simulink model "UPS_3level_Ttype_Inverter_simplified_ctrl"  (R2012b)
settings: Solver=ode4  StartTime=0.0  StopTime=Tfinal  FixedStep=Ts  MaxStep=1e-5  RelTol=1e-3
values from neighbouring files (symbols this model uses):
  Ts = 1/(1*1e6)    (= 1e-06)    [Run.m]
  Vd = 720    [Run.m]
  VSI = rmfield(VSI, {'IF1', 'IF2', 'FLUXlin1', 'FLUXlin2',      'FLUXnonlin1', 'FLUXnonlin2', 'Lfnonlin'})    [Run.m]
undefined symbols (not defined in the file or in its folder): ADC, CTRL, DiscIntNeverNeededParam, PR, S, UPS
libraries: powerlib x113, simulink_extras x11, powerlib_extras x11, simulink x3
(part 2 of 3)

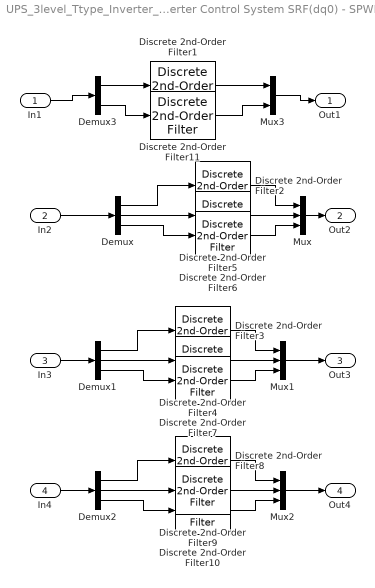
== system UPS_3level_Ttype_Inverter_simplified_ctrl/Output Inverter Control System SRF(dq0) - SPWM /input filter1 ==
  In1 : Inport
  In2 : Inport  Port=2
  In3 : Inport  Port=3
  In4 : Inport  Port=4
  Demux : Demux  Outputs=3
  Demux1 : Demux  Outputs=3
  Demux2 : Demux  Outputs=3
  Demux3 : Demux  Outputs=2
  Discrete 2nd-Order Filter1 : powerlib_extras/Discrete  Control Blocks/Discrete  2nd-Order Filter  FilterType=Lowpass  Fo=25000  Zeta=0.89  Ts=Ts  Initialize=off  Vac_Init=[0.8 -25 60]  Vdc_Init=-0.4  PlotResponse=off  param1=[1 500 1]
  Discrete 2nd-Order Filter{2..10} (9 alike) : powerlib_extras/Discrete  Control Blocks/Discrete  2nd-Order Filter  FilterType=Lowpass  Fo=25e3  Zeta=0.89  Ts=Ts  Initialize=off  Vac_Init=[0.8 -25 60]  Vdc_Init=-0.4  PlotResponse=off  param1=[1 500 1]
  Discrete 2nd-Order Filter11 : powerlib_extras/Discrete  Control Blocks/Discrete  2nd-Order Filter  FilterType=Lowpass  Fo=25000  Zeta=0.89  Ts=Ts  Initialize=off  Vac_Init=[0.8 -25 60]  Vdc_Init=-0.4  PlotResponse=off  param1=[1 500 1]
  Mux : Mux  Inputs=3
  Mux1 : Mux  Inputs=3
  Mux2 : Mux  Inputs=3
  Mux3 : Mux  Inputs=2
  Out1 : Outport
  Out2 : Outport  Port=2
  Out3 : Outport  Port=3
  Out4 : Outport  Port=4
  wires:
  Demux/3 -> Discrete 2nd-Order Filter6/1
  In2/1 -> Demux/1
  Mux/1 -> Out2/1
  Demux/1 -> Discrete 2nd-Order Filter2/1
  Demux/2 -> Discrete 2nd-Order Filter5/1
  Discrete 2nd-Order Filter5/1 -> Mux/2
  Discrete 2nd-Order Filter6/1 -> Mux/3
  Discrete 2nd-Order Filter2/1 -> Mux/1
  Demux1/3 -> Discrete 2nd-Order Filter7/1
  Demux1/1 -> Discrete 2nd-Order Filter3/1
  Demux1/2 -> Discrete 2nd-Order Filter4/1
  Discrete 2nd-Order Filter4/1 -> Mux1/2
  Discrete 2nd-Order Filter7/1 -> Mux1/3
  Discrete 2nd-Order Filter3/1 -> Mux1/1
  Demux2/3 -> Discrete 2nd-Order Filter10/1
  Demux2/1 -> Discrete 2nd-Order Filter8/1
  Demux2/2 -> Discrete 2nd-Order Filter9/1
  Discrete 2nd-Order Filter9/1 -> Mux2/2
  Discrete 2nd-Order Filter10/1 -> Mux2/3
  Discrete 2nd-Order Filter8/1 -> Mux2/1
  Mux2/1 -> Out4/1
  Mux1/1 -> Out3/1
  In3/1 -> Demux1/1
  In4/1 -> Demux2/1
  Demux3/2 -> Discrete 2nd-Order Filter11/1
  Demux3/1 -> Discrete 2nd-Order Filter1/1
  Discrete 2nd-Order Filter1/1 -> Mux3/1
  Discrete 2nd-Order Filter11/1 -> Mux3/2
  Mux3/1 -> Out1/1
  In1/1 -> Demux3/1

== system UPS_3level_Ttype_Inverter_simplified_ctrl/Output filter (Cf2, Lf2)/2phasM1 ==
  Constant2 : Constant  Value=UPS.Lfnonlin
  Data Type Conversion2 : DataTypeConversion  OutDataTypeStr=boolean  SaturateOnIntegerOverflow=on  RndMeth=Zero
  Discrete-Time Integrator : DiscreteIntegrator  gainval=1  SampleTime=Ts  ICPrevOutput=DiscIntNeverNeededParam  ICPrevScaledInput=DiscIntNeverNeededParam
  Lookup Table : Lookup  InputValues=VSI.FLUXnonlin  Table=VSI.IF
  Lookup Table1 : Lookup  InputValues=VSI.FLUXlin  Table=VSI.IF
  Switch2 : Switch  Threshold=1
  if : powerlib/Electrical Sources/Controlled Current Source  Initialize=on  Source_Type=AC  Amplitude=0  Phase=0  Frequency=0  Measurements=None
  vf : powerlib/Measurements/Voltage Measurement  PhasorSimulation=off  OutputType=Complex  PSBequivalent=0
  x : PMIOPort  Port=1  Side=Left
  y : PMIOPort  Port=2  Side=Right
  wires:
  vf/1 -> Discrete-Time Integrator/1
  Discrete-Time Integrator/1 -> Lookup Table/1, Lookup Table1/1
  Data Type Conversion2/1 -> Switch2/2
  Constant2/1 -> Data Type Conversion2/1
  Lookup Table1/1 -> Switch2/3
  Lookup Table/1 -> Switch2/1
  Switch2/1 -> if/1
  connections:
  if/RConn1 -- y/RConn1 -- vf/LConn2
  x/RConn1 -- vf/LConn1 -- if/LConn1

== system UPS_3level_Ttype_Inverter_simplified_ctrl/Output filter (Cf2, Lf2)/2phasM2 ==
  Constant2 : Constant  Value=UPS.Lfnonlin
  Data Type Conversion2 : DataTypeConversion  OutDataTypeStr=boolean  SaturateOnIntegerOverflow=on  RndMeth=Zero
  Discrete-Time Integrator : DiscreteIntegrator  gainval=1  SampleTime=Ts  ICPrevOutput=DiscIntNeverNeededParam  ICPrevScaledInput=DiscIntNeverNeededParam
  Lookup Table : Lookup  InputValues=VSI.FLUXnonlin  Table=VSI.IF
  Lookup Table1 : Lookup  InputValues=VSI.FLUXlin  Table=VSI.IF
  Switch2 : Switch  Threshold=1
  if : powerlib/Electrical Sources/Controlled Current Source  Initialize=on  Source_Type=AC  Amplitude=0  Phase=0  Frequency=0  Measurements=None
  vf : powerlib/Measurements/Voltage Measurement  PhasorSimulation=off  OutputType=Complex  PSBequivalent=0
  x : PMIOPort  Port=1  Side=Left
  y : PMIOPort  Port=2  Side=Right
  wires:
  vf/1 -> Discrete-Time Integrator/1
  Discrete-Time Integrator/1 -> Lookup Table/1, Lookup Table1/1
  Data Type Conversion2/1 -> Switch2/2
  Constant2/1 -> Data Type Conversion2/1
  Lookup Table1/1 -> Switch2/3
  Lookup Table/1 -> Switch2/1
  Switch2/1 -> if/1
  connections:
  if/RConn1 -- y/RConn1 -- vf/LConn2
  x/RConn1 -- vf/LConn1 -- if/LConn1

== system UPS_3level_Ttype_Inverter_simplified_ctrl/Output filter (Cf2, Lf2)/2phasM8 ==
  Constant2 : Constant  Value=UPS.Lfnonlin
  Data Type Conversion2 : DataTypeConversion  OutDataTypeStr=boolean  SaturateOnIntegerOverflow=on  RndMeth=Zero
  Discrete-Time Integrator : DiscreteIntegrator  gainval=1  SampleTime=Ts  ICPrevOutput=DiscIntNeverNeededParam  ICPrevScaledInput=DiscIntNeverNeededParam
  Lookup Table : Lookup  InputValues=VSI.FLUXnonlin  Table=VSI.IF
  Lookup Table1 : Lookup  InputValues=VSI.FLUXlin  Table=VSI.IF
  Switch2 : Switch  Threshold=1
  if : powerlib/Electrical Sources/Controlled Current Source  Initialize=on  Source_Type=AC  Amplitude=0  Phase=0  Frequency=0  Measurements=None
  vf : powerlib/Measurements/Voltage Measurement  PhasorSimulation=off  OutputType=Complex  PSBequivalent=0
  x : PMIOPort  Port=1  Side=Left
  y : PMIOPort  Port=2  Side=Right
  wires:
  vf/1 -> Discrete-Time Integrator/1
  Discrete-Time Integrator/1 -> Lookup Table/1, Lookup Table1/1
  Data Type Conversion2/1 -> Switch2/2
  Constant2/1 -> Data Type Conversion2/1
  Lookup Table1/1 -> Switch2/3
  Lookup Table/1 -> Switch2/1
  Switch2/1 -> if/1
  connections:
  if/RConn1 -- y/RConn1 -- vf/LConn2
  x/RConn1 -- vf/LConn1 -- if/LConn1

== system UPS_3level_Ttype_Inverter_simplified_ctrl/Output Inverter Control System SRF(dq0) - SPWM /3p PLL/va, vb ==
  Vm* [pu] : Inport
  "wrt* [deg] " : Inport  Port=2
  va* = Vm*cos(wrt)* : Subsystem
  vb* = Vm*sin(wrt)* : Subsystem
  cos(wrt)* : Outport
  sin(wrt)* : Outport  Port=2
  wires:
  Vm* [pu]/1 -> va* = Vm*cos(wrt)*/1(Vm [pu]), vb* = Vm*sin(wrt)*/1(Vm [pu])
  va* = Vm*cos(wrt)*/1(va) -> cos(wrt)*/1
  vb* = Vm*sin(wrt)*/1(vb) -> sin(wrt)*/1
  "wrt* [deg] "/1 -> vb* = Vm*sin(wrt)*/2(wrt [deg]), va* = Vm*cos(wrt)*/2(wrt [deg])

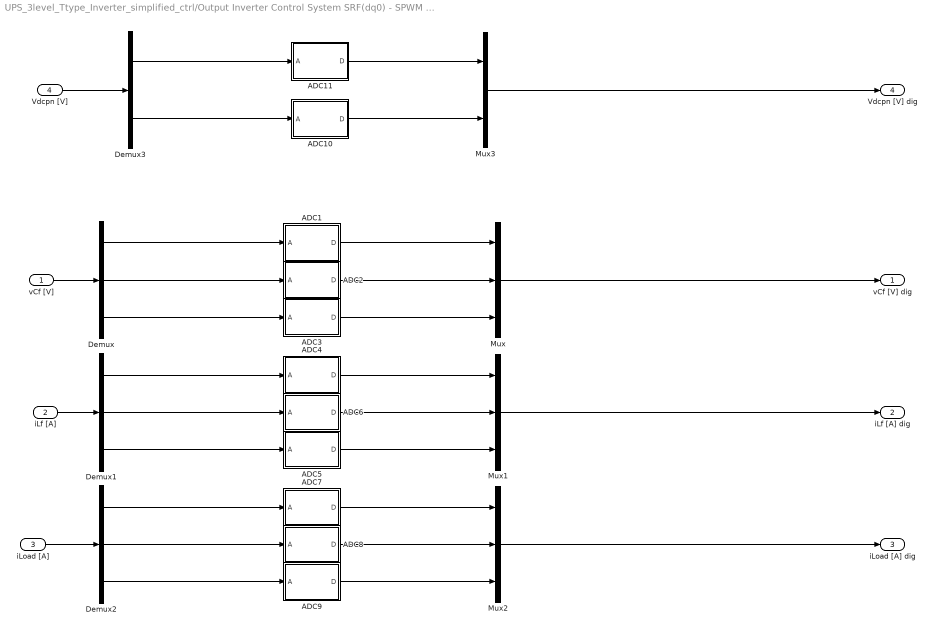
== system UPS_3level_Ttype_Inverter_simplified_ctrl/Output Inverter Control System SRF(dq0) - SPWM /SPWM (Treg)2/ ADC System (Tinp//2) ==
  vCf [V] : Inport
  iLf [A] : Inport  Port=2
  iLoad [A] : Inport  Port=3
  Vdcpn [V] : Inport  Port=4
  ADC1 : Subsystem
  ADC10 : Subsystem
  ADC11 : Subsystem
  ADC2 : Subsystem
  ADC3 : Subsystem
  ADC4 : Subsystem
  ADC5 : Subsystem
  ADC6 : Subsystem
  ADC7 : Subsystem
  ADC8 : Subsystem
  ADC9 : Subsystem
  Demux : Demux  Outputs=3
  Demux1 : Demux  Outputs=3
  Demux2 : Demux  Outputs=3
  Demux3 : Demux  Outputs=2
  Mux : Mux  Inputs=3
  Mux1 : Mux  Inputs=3
  Mux2 : Mux  Inputs=3
  Mux3 : Mux  Inputs=2
  vCf [V] dig : Outport
  iLf [A] dig : Outport  Port=2
  iLoad [A] dig : Outport  Port=3
  Vdcpn [V] dig : Outport  Port=4
  wires:
  Demux/1 -> ADC1/1(A)
  Demux/2 -> ADC2/1(A)
  Demux/3 -> ADC3/1(A)
  ADC1/1(D) -> Mux/1
  ADC2/1(D) -> Mux/2
  ADC3/1(D) -> Mux/3
  Demux1/1 -> ADC4/1(A)
  Demux1/2 -> ADC6/1(A)
  Demux1/3 -> ADC5/1(A)
  ADC4/1(D) -> Mux1/1
  ADC6/1(D) -> Mux1/2
  ADC5/1(D) -> Mux1/3
  Demux2/1 -> ADC7/1(A)
  Demux2/2 -> ADC8/1(A)
  Demux2/3 -> ADC9/1(A)
  ADC7/1(D) -> Mux2/1
  ADC8/1(D) -> Mux2/2
  ADC9/1(D) -> Mux2/3
  vCf [V]/1 -> Demux/1
  iLf [A]/1 -> Demux1/1
  iLoad [A]/1 -> Demux2/1
  Mux/1 -> vCf [V] dig/1
  Mux1/1 -> iLf [A] dig/1
  Mux2/1 -> iLoad [A] dig/1
  Mux3/1 -> Vdcpn [V] dig/1
  ADC10/1(D) -> Mux3/2
  Demux3/2 -> ADC10/1(A)
  Demux3/1 -> ADC11/1(A)
  ADC11/1(D) -> Mux3/1
  Vdcpn [V]/1 -> Demux3/1

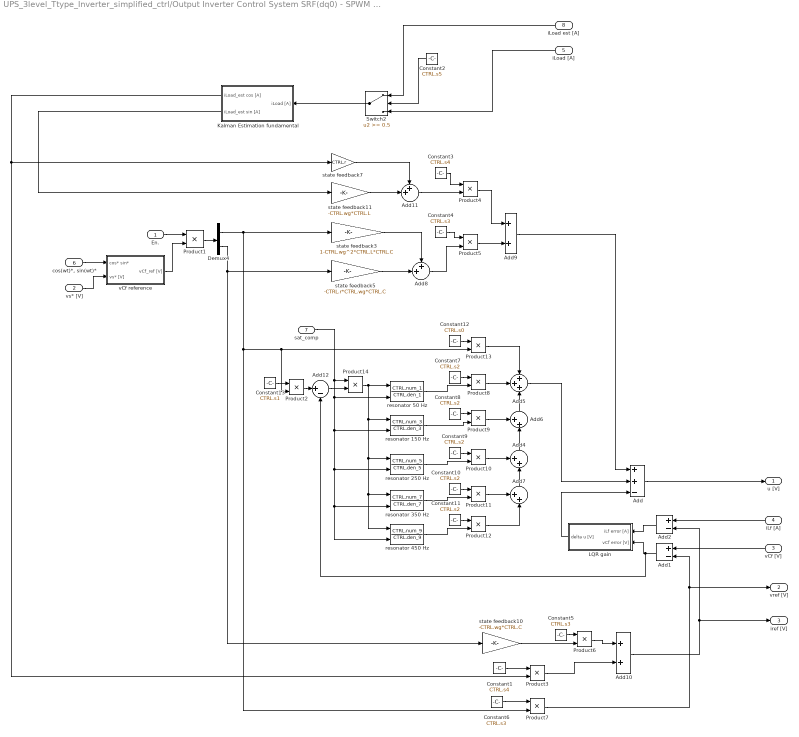
== system UPS_3level_Ttype_Inverter_simplified_ctrl/Output Inverter Control System SRF(dq0) - SPWM /SPWM (Treg)2/controller ph a1 ==
  En. : Inport
  vs* [V] : Inport  Port=2
  vCf [V] : Inport  Port=3
  iLf [A] : Inport  Port=4
  iLoad [A] : Inport  Port=5
  "cos(wt)*, sin(wt)*" : Inport  Port=6
  sat_comp : Inport  Port=7
  iLoad est [A] : Inport  Port=8
  Add : Sum  Inputs=++-
  Add1 : Sum  Inputs=+-
  Add10 : Sum
  Add{4,6..8,11} (5 alike) : Sum  Inputs=++|
  Add12 : Sum  Inputs=|+-
  Add2 : Sum  Inputs=+-
  Add5 : Sum  Inputs=+++
  Add9 : Sum
  Constant1 : Constant  Value=CTRL.s4
  Constant{7..11} (5 alike) : Constant  Value=CTRL.s2
  Constant12 : Constant  Value=CTRL.s0
  Constant13 : Constant  Value=CTRL.s1
  Constant2 : Constant  Value=CTRL.s5
  Constant3 : Constant  Value=CTRL.s4
  Constant4 : Constant  Value=CTRL.s3
  Constant5 : Constant  Value=CTRL.s3
  Constant6 : Constant  Value=CTRL.s3
  Demux4 : Demux  Outputs=2
  Kalman Estimation fundamental : Subsystem
  LQR gain : Subsystem
  Product{1..14} (14 alike) : Product  RndMeth=Zero
  Switch2 : Switch  Threshold=0.5
  resonator 150 Hz : DiscreteTransferFcn  Numerator=CTRL.num_3  Denominator=CTRL.den_3  ExternalReset=Falling
      settings: InputPortMap=u0,r7
  resonator 250 Hz : DiscreteTransferFcn  Numerator=CTRL.num_5  Denominator=CTRL.den_5  ExternalReset=Falling
      settings: InputPortMap=u0,r7
  resonator 350 Hz : DiscreteTransferFcn  Numerator=CTRL.num_7  Denominator=CTRL.den_7  ExternalReset=Falling
      settings: InputPortMap=u0,r7
  resonator 450 Hz : DiscreteTransferFcn  Numerator=CTRL.num_9  Denominator=CTRL.den_9  ExternalReset=Falling
      settings: InputPortMap=u0,r7
  resonator 50 Hz : DiscreteTransferFcn  Numerator=CTRL.num_1  Denominator=CTRL.den_1  ExternalReset=Falling
      settings: InputPortMap=u0,r7
  state feedback10 : Gain  Gain=-CTRL.wg*CTRL.C
  state feedback11 : Gain  Gain=-CTRL.wg*CTRL.L
  state feedback3 : Gain  Gain=1-CTRL.wg^2*CTRL.L*CTRL.C
  state feedback5 : Gain  Gain=-CTRL.r*CTRL.wg*CTRL.C
  state feedback7 : Gain  Gain=CTRL.r
  vCf reference : Subsystem
  u [V] : Outport
  vref [V] : Outport  Port=2
  iref [V] : Outport  Port=3
  wires:
  vs* [V]/1 -> vCf reference/2(vs* [V])
  "cos(wt)*, sin(wt)*"/1 -> vCf reference/1(cos* sin*)
  En./1 -> Product1/1
  vCf reference/1(vCf_ref [V]) -> Product1/2
  Add2/1 -> LQR gain/1(iLf error [A])
  LQR gain/1(delta u [V]) -> Add/3
  Product1/1 -> Demux4/1
  iLf [A]/1 -> Add2/1
  Add/1 -> u [V]/1
  vCf [V]/1 -> Add1/1
  Add10/1 -> iref [V]/1, Add2/2
  state feedback10/1 -> Product6/2
  Kalman Estimation fundamental/1(iLoad_est cos [A]) -> Product3/2, state feedback7/1
  Demux4/2 -> state feedback5/1, state feedback10/1
  Demux4/1 -> state feedback3/1, Product2/2, Product13/2, Product7/2
  Kalman Estimation fundamental/2(iLoad_est sin [A]) -> state feedback11/1
  Add9/1 -> Add/1
  Add11/1 -> Product4/2
  state feedback7/1 -> Add11/1
  state feedback5/1 -> Add8/2
  state feedback11/1 -> Add11/2
  state feedback3/1 -> Add8/1
  Add8/1 -> Product5/2
  Add5/1 -> Add/2
  Add7/1 -> Add4/2
  Add4/1 -> Add6/2
  Add6/1 -> Add5/3
  Product14/1 -> resonator 450 Hz/1, resonator 350 Hz/1, resonator 250 Hz/1, resonator 150 Hz/1, resonator 50 Hz/1
  Add1/1 -> Add12/2, LQR gain/2(vCf error [V])
  Constant2/1 -> Switch2/2
  Switch2/1 -> Kalman Estimation fundamental/1(iLoad [A])
  iLoad est [A]/1 -> Switch2/1
  iLoad [A]/1 -> Switch2/3
  Constant1/1 -> Product3/1
  Product3/1 -> Add10/2
  Constant3/1 -> Product4/1
  Product4/1 -> Add9/1
  Constant4/1 -> Product5/1
  Product5/1 -> Add9/2
  Constant5/1 -> Product6/1
  Product6/1 -> Add10/1
  Constant6/1 -> Product7/1
  Product7/1 -> Add1/2, vref [V]/1
  Constant7/1 -> Product8/1
  Constant8/1 -> Product9/1
  Constant9/1 -> Product10/1
  Constant10/1 -> Product11/1
  Constant11/1 -> Product12/1
  Product8/1 -> Add5/2
  Product9/1 -> Add6/1
  Product10/1 -> Add4/1
  Product11/1 -> Add7/1
  Product12/1 -> Add7/2
  resonator 450 Hz/1 -> Product12/2
  resonator 50 Hz/1 -> Product8/2
  resonator 150 Hz/1 -> Product9/2
  resonator 250 Hz/1 -> Product10/2
  resonator 350 Hz/1 -> Product11/2
  Constant12/1 -> Product13/1
  Product13/1 -> Add5/1
  Constant13/1 -> Product2/1
  Product2/1 -> Add12/1
  Add12/1 -> Product14/2
  sat_comp/1 -> Product14/1, resonator 450 Hz/2, resonator 350 Hz/2, resonator 250 Hz/2, resonator 150 Hz/2, resonator 50 Hz/2

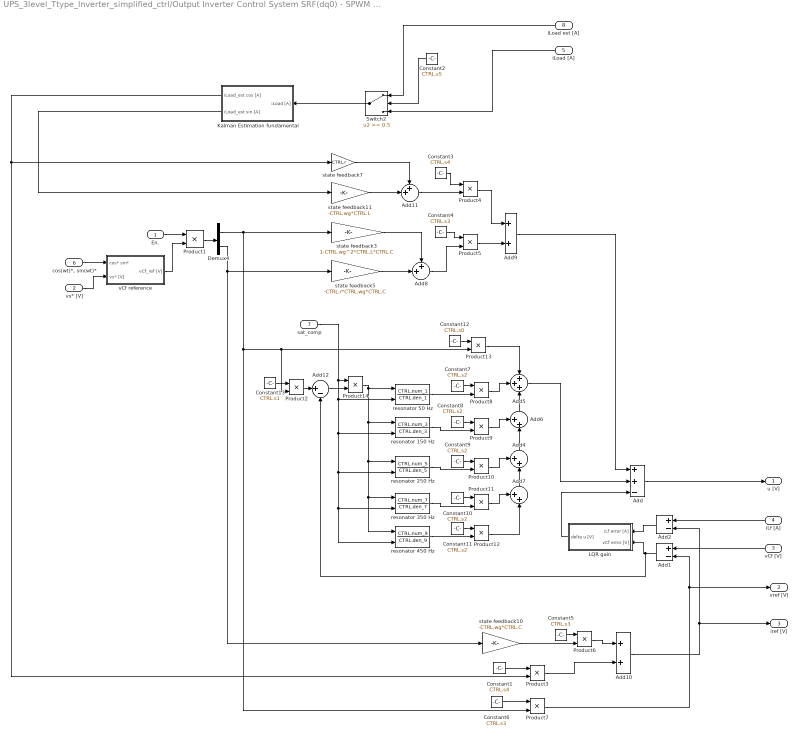
== system UPS_3level_Ttype_Inverter_simplified_ctrl/Output Inverter Control System SRF(dq0) - SPWM /SPWM (Treg)2/controller ph a2 ==
  En. : Inport
  vs* [V] : Inport  Port=2
  vCf [V] : Inport  Port=3
  iLf [A] : Inport  Port=4
  iLoad [A] : Inport  Port=5
  "cos(wt)*, sin(wt)*" : Inport  Port=6
  sat_comp : Inport  Port=7
  iLoad est [A] : Inport  Port=8
  Add : Sum  Inputs=++-
  Add1 : Sum  Inputs=+-
  Add10 : Sum
  Add{4,6..8,11} (5 alike) : Sum  Inputs=++|
  Add12 : Sum  Inputs=|+-
  Add2 : Sum  Inputs=+-
  Add5 : Sum  Inputs=+++
  Add9 : Sum
  Constant1 : Constant  Value=CTRL.s4
  Constant{7..11} (5 alike) : Constant  Value=CTRL.s2
  Constant12 : Constant  Value=CTRL.s0
  Constant13 : Constant  Value=CTRL.s1
  Constant2 : Constant  Value=CTRL.s5
  Constant3 : Constant  Value=CTRL.s4
  Constant4 : Constant  Value=CTRL.s3
  Constant5 : Constant  Value=CTRL.s3
  Constant6 : Constant  Value=CTRL.s3
  Demux4 : Demux  Outputs=2
  Kalman Estimation fundamental : Subsystem
  LQR gain : Subsystem
  Product{1..14} (14 alike) : Product  RndMeth=Zero
  Switch2 : Switch  Threshold=0.5
  resonator 150 Hz : DiscreteTransferFcn  Numerator=CTRL.num_3  Denominator=CTRL.den_3  ExternalReset=Falling
      settings: InputPortMap=u0,r7
  resonator 250 Hz : DiscreteTransferFcn  Numerator=CTRL.num_5  Denominator=CTRL.den_5  ExternalReset=Falling
      settings: InputPortMap=u0,r7
  resonator 350 Hz : DiscreteTransferFcn  Numerator=CTRL.num_7  Denominator=CTRL.den_7  ExternalReset=Falling
      settings: InputPortMap=u0,r7
  resonator 450 Hz : DiscreteTransferFcn  Numerator=CTRL.num_9  Denominator=CTRL.den_9  ExternalReset=Falling
      settings: InputPortMap=u0,r7
  resonator 50 Hz : DiscreteTransferFcn  Numerator=CTRL.num_1  Denominator=CTRL.den_1  ExternalReset=Falling
      settings: InputPortMap=u0,r7
  state feedback10 : Gain  Gain=-CTRL.wg*CTRL.C
  state feedback11 : Gain  Gain=-CTRL.wg*CTRL.L
  state feedback3 : Gain  Gain=1-CTRL.wg^2*CTRL.L*CTRL.C
  state feedback5 : Gain  Gain=-CTRL.r*CTRL.wg*CTRL.C
  state feedback7 : Gain  Gain=CTRL.r
  vCf reference : Subsystem
  u [V] : Outport
  vref [V] : Outport  Port=2
  iref [V] : Outport  Port=3
  wires:
  Add12/1 -> Product14/2
  sat_comp/1 -> resonator 450 Hz/2, resonator 350 Hz/2, resonator 250 Hz/2, resonator 150 Hz/2, resonator 50 Hz/2, Product14/1
  Product2/1 -> Add12/1
  Constant13/1 -> Product2/1
  Product13/1 -> Add5/1
  Constant12/1 -> Product13/1
  resonator 350 Hz/1 -> Product11/2
  resonator 250 Hz/1 -> Product10/2
  resonator 150 Hz/1 -> Product9/2
  resonator 50 Hz/1 -> Product8/2
  resonator 450 Hz/1 -> Product12/2
  Product12/1 -> Add7/2
  Product11/1 -> Add7/1
  Product10/1 -> Add4/1
  Product9/1 -> Add6/1
  Product8/1 -> Add5/2
  Constant11/1 -> Product12/1
  Constant10/1 -> Product11/1
  Constant9/1 -> Product10/1
  Constant8/1 -> Product9/1
  Constant7/1 -> Product8/1
  Product7/1 -> vref [V]/1, Add1/2
  Constant6/1 -> Product7/1
  Product6/1 -> Add10/1
  Constant5/1 -> Product6/1
  Product5/1 -> Add9/2
  Constant4/1 -> Product5/1
  Product4/1 -> Add9/1
  Constant3/1 -> Product4/1
  Product3/1 -> Add10/2
  Constant1/1 -> Product3/1
  iLoad [A]/1 -> Switch2/3
  iLoad est [A]/1 -> Switch2/1
  Switch2/1 -> Kalman Estimation fundamental/1(iLoad [A])
  Constant2/1 -> Switch2/2
  Add1/1 -> LQR gain/2(vCf error [V]), Add12/2
  Product14/1 -> resonator 50 Hz/1, resonator 150 Hz/1, resonator 250 Hz/1, resonator 350 Hz/1, resonator 450 Hz/1
  Add6/1 -> Add5/3
  Add4/1 -> Add6/2
  Add7/1 -> Add4/2
  Add5/1 -> Add/2
  Add8/1 -> Product5/2
  state feedback3/1 -> Add8/1
  state feedback11/1 -> Add11/2
  state feedback5/1 -> Add8/2
  state feedback7/1 -> Add11/1
  Add11/1 -> Product4/2
  Add9/1 -> Add/1
  Kalman Estimation fundamental/2(iLoad_est sin [A]) -> state feedback11/1
  Demux4/1 -> Product7/2, Product13/2, Product2/2, state feedback3/1
  Demux4/2 -> state feedback10/1, state feedback5/1
  Kalman Estimation fundamental/1(iLoad_est cos [A]) -> state feedback7/1, Product3/2
  state feedback10/1 -> Product6/2
  Add10/1 -> iref [V]/1, Add2/2
  vCf [V]/1 -> Add1/1
  Add/1 -> u [V]/1
  iLf [A]/1 -> Add2/1
  Product1/1 -> Demux4/1
  LQR gain/1(delta u [V]) -> Add/3
  Add2/1 -> LQR gain/1(iLf error [A])
  vCf reference/1(vCf_ref [V]) -> Product1/2
  En./1 -> Product1/1
  "cos(wt)*, sin(wt)*"/1 -> vCf reference/1(cos* sin*)
  vs* [V]/1 -> vCf reference/2(vs* [V])

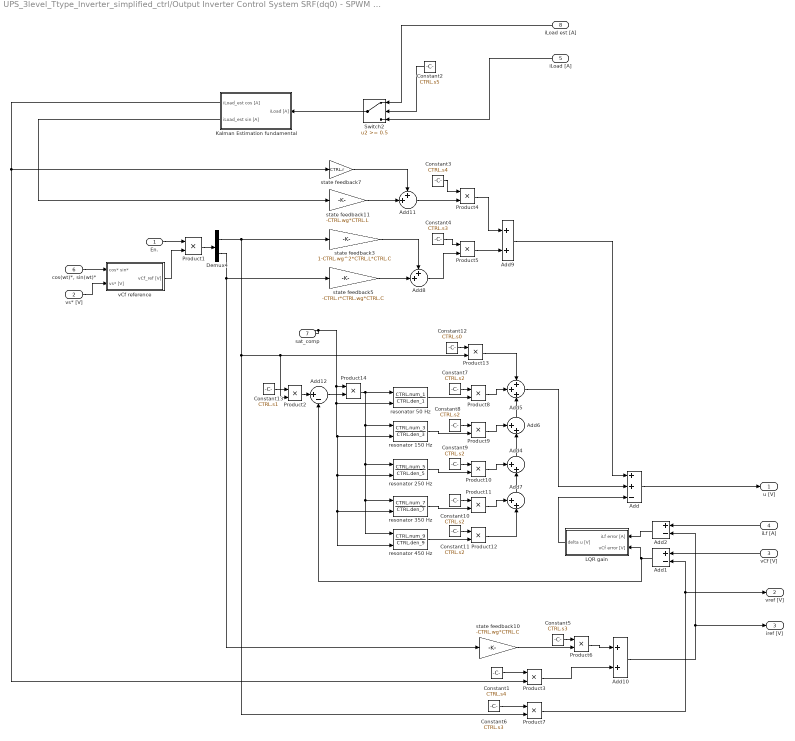
== system UPS_3level_Ttype_Inverter_simplified_ctrl/Output Inverter Control System SRF(dq0) - SPWM /SPWM (Treg)2/controller ph a3 ==
  En. : Inport
  vs* [V] : Inport  Port=2
  vCf [V] : Inport  Port=3
  iLf [A] : Inport  Port=4
  iLoad [A] : Inport  Port=5
  "cos(wt)*, sin(wt)*" : Inport  Port=6
  sat_comp : Inport  Port=7
  iLoad est [A] : Inport  Port=8
  Add : Sum  Inputs=++-
  Add1 : Sum  Inputs=+-
  Add10 : Sum
  Add{4,6..8,11} (5 alike) : Sum  Inputs=++|
  Add12 : Sum  Inputs=|+-
  Add2 : Sum  Inputs=+-
  Add5 : Sum  Inputs=+++
  Add9 : Sum
  Constant1 : Constant  Value=CTRL.s4
  Constant{7..11} (5 alike) : Constant  Value=CTRL.s2
  Constant12 : Constant  Value=CTRL.s0
  Constant13 : Constant  Value=CTRL.s1
  Constant2 : Constant  Value=CTRL.s5
  Constant3 : Constant  Value=CTRL.s4
  Constant4 : Constant  Value=CTRL.s3
  Constant5 : Constant  Value=CTRL.s3
  Constant6 : Constant  Value=CTRL.s3
  Demux4 : Demux  Outputs=2
  Kalman Estimation fundamental : Subsystem
  LQR gain : Subsystem
  Product{1..14} (14 alike) : Product  RndMeth=Zero
  Switch2 : Switch  Threshold=0.5
  resonator 150 Hz : DiscreteTransferFcn  Numerator=CTRL.num_3  Denominator=CTRL.den_3  ExternalReset=Falling
      settings: InputPortMap=u0,r7
  resonator 250 Hz : DiscreteTransferFcn  Numerator=CTRL.num_5  Denominator=CTRL.den_5  ExternalReset=Falling
      settings: InputPortMap=u0,r7
  resonator 350 Hz : DiscreteTransferFcn  Numerator=CTRL.num_7  Denominator=CTRL.den_7  ExternalReset=Falling
      settings: InputPortMap=u0,r7
  resonator 450 Hz : DiscreteTransferFcn  Numerator=CTRL.num_9  Denominator=CTRL.den_9  ExternalReset=Falling
      settings: InputPortMap=u0,r7
  resonator 50 Hz : DiscreteTransferFcn  Numerator=CTRL.num_1  Denominator=CTRL.den_1  ExternalReset=Falling
      settings: InputPortMap=u0,r7
  state feedback10 : Gain  Gain=-CTRL.wg*CTRL.C
  state feedback11 : Gain  Gain=-CTRL.wg*CTRL.L
  state feedback3 : Gain  Gain=1-CTRL.wg^2*CTRL.L*CTRL.C
  state feedback5 : Gain  Gain=-CTRL.r*CTRL.wg*CTRL.C
  state feedback7 : Gain  Gain=CTRL.r
  vCf reference : Subsystem
  u [V] : Outport
  vref [V] : Outport  Port=2
  iref [V] : Outport  Port=3
  wires:
  vs* [V]/1 -> vCf reference/2(vs* [V])
  "cos(wt)*, sin(wt)*"/1 -> vCf reference/1(cos* sin*)
  En./1 -> Product1/1
  vCf reference/1(vCf_ref [V]) -> Product1/2
  Add2/1 -> LQR gain/1(iLf error [A])
  LQR gain/1(delta u [V]) -> Add/3
  Product1/1 -> Demux4/1
  iLf [A]/1 -> Add2/1
  Add/1 -> u [V]/1
  vCf [V]/1 -> Add1/1
  Add10/1 -> iref [V]/1, Add2/2
  state feedback10/1 -> Product6/2
  Kalman Estimation fundamental/1(iLoad_est cos [A]) -> Product3/2, state feedback7/1
  Demux4/2 -> state feedback5/1, state feedback10/1
  Demux4/1 -> state feedback3/1, Product2/2, Product13/2, Product7/2
  Kalman Estimation fundamental/2(iLoad_est sin [A]) -> state feedback11/1
  Add9/1 -> Add/1
  Add11/1 -> Product4/2
  state feedback7/1 -> Add11/1
  state feedback5/1 -> Add8/2
  state feedback11/1 -> Add11/2
  state feedback3/1 -> Add8/1
  Add8/1 -> Product5/2
  Add5/1 -> Add/2
  Add7/1 -> Add4/2
  Add4/1 -> Add6/2
  Add6/1 -> Add5/3
  Product14/1 -> resonator 450 Hz/1, resonator 350 Hz/1, resonator 250 Hz/1, resonator 150 Hz/1, resonator 50 Hz/1
  Add1/1 -> Add12/2, LQR gain/2(vCf error [V])
  Constant2/1 -> Switch2/2
  Switch2/1 -> Kalman Estimation fundamental/1(iLoad [A])
  iLoad est [A]/1 -> Switch2/1
  iLoad [A]/1 -> Switch2/3
  Constant1/1 -> Product3/1
  Product3/1 -> Add10/2
  Constant3/1 -> Product4/1
  Product4/1 -> Add9/1
  Constant4/1 -> Product5/1
  Product5/1 -> Add9/2
  Constant5/1 -> Product6/1
  Product6/1 -> Add10/1
  Constant6/1 -> Product7/1
  Product7/1 -> Add1/2, vref [V]/1
  Constant7/1 -> Product8/1
  Constant8/1 -> Product9/1
  Constant9/1 -> Product10/1
  Constant10/1 -> Product11/1
  Constant11/1 -> Product12/1
  Product8/1 -> Add5/2
  Product9/1 -> Add6/1
  Product10/1 -> Add4/1
  Product11/1 -> Add7/1
  Product12/1 -> Add7/2
  resonator 450 Hz/1 -> Product12/2
  resonator 50 Hz/1 -> Product8/2
  resonator 150 Hz/1 -> Product9/2
  resonator 250 Hz/1 -> Product10/2
  resonator 350 Hz/1 -> Product11/2
  Constant12/1 -> Product13/1
  Product13/1 -> Add5/1
  Constant13/1 -> Product2/1
  Product2/1 -> Add12/1
  sat_comp/1 -> resonator 450 Hz/2, resonator 350 Hz/2, resonator 250 Hz/2, resonator 150 Hz/2, resonator 50 Hz/2, Product14/1
  Add12/1 -> Product14/2

== system UPS_3level_Ttype_Inverter_simplified_ctrl/Output Inverter Control System SRF(dq0) - SPWM /SPWM (Treg)2/iLoad estimator ==
  iLf [A] : Inport
  vCf [V] : Inport  Port=2
  Add : Sum  Inputs=+-
  Add1 : Sum  Inputs=+-
  Discrete Transfer Fcn7 : DiscreteTransferFcn  Numerator=CTRL.num_lp  Denominator=CTRL.den_lp
  Gain1 : Gain  Gain=VSI.Cf/VSI.Treg
  Unit Delay : UnitDelay  SampleTime=-1
  iLoad_est [A] : Outport
  wires:
  Discrete Transfer Fcn7/1 -> iLoad_est [A]/1
  iLf [A]/1 -> Add/1
  Add1/1 -> Gain1/1
  Unit Delay/1 -> Add1/2
  vCf [V]/1 -> Add1/1, Unit Delay/1
  Gain1/1 -> Add/2
  Add/1 -> Discrete Transfer Fcn7/1

== system UPS_3level_Ttype_Inverter_simplified_ctrl/Output Inverter Control System SRF(dq0) - SPWM /SPWM (Treg)2/iLoad estimator1 ==
  iLf [A] : Inport
  vCf [V] : Inport  Port=2
  Add : Sum  Inputs=+-
  Add1 : Sum  Inputs=+-
  Discrete Transfer Fcn7 : DiscreteTransferFcn  Numerator=CTRL.num_lp  Denominator=CTRL.den_lp
  Gain1 : Gain  Gain=VSI.Cf/VSI.Treg
  Unit Delay : UnitDelay  SampleTime=-1
  iLoad_est [A] : Outport
  wires:
  Add/1 -> Discrete Transfer Fcn7/1
  Gain1/1 -> Add/2
  vCf [V]/1 -> Unit Delay/1, Add1/1
  Unit Delay/1 -> Add1/2
  Add1/1 -> Gain1/1
  iLf [A]/1 -> Add/1
  Discrete Transfer Fcn7/1 -> iLoad_est [A]/1

== system UPS_3level_Ttype_Inverter_simplified_ctrl/Output Inverter Control System SRF(dq0) - SPWM /SPWM (Treg)2/iLoad estimator2 ==
  iLf [A] : Inport
  vCf [V] : Inport  Port=2
  Add : Sum  Inputs=+-
  Add1 : Sum  Inputs=+-
  Discrete Transfer Fcn7 : DiscreteTransferFcn  Numerator=CTRL.num_lp  Denominator=CTRL.den_lp
  Gain1 : Gain  Gain=VSI.Cf/VSI.Treg
  Unit Delay : UnitDelay  SampleTime=-1
  iLoad_est [A] : Outport
  wires:
  Discrete Transfer Fcn7/1 -> iLoad_est [A]/1
  iLf [A]/1 -> Add/1
  Add1/1 -> Gain1/1
  Unit Delay/1 -> Add1/2
  vCf [V]/1 -> Add1/1, Unit Delay/1
  Gain1/1 -> Add/2
  Add/1 -> Discrete Transfer Fcn7/1

== system UPS_3level_Ttype_Inverter_simplified_ctrl/Output Inverter Control System SRF(dq0) - SPWM /SPWM (Treg)2/phase a signals ==
  vCf [V] : Inport
  iLf [A] : Inport  Port=2
  iLoad [A] : Inport  Port=3
  cos sin : Inport  Port=4
  Demux : Demux  Outputs=3
  Demux1 : Demux  Outputs=3
  Demux2 : Demux  Outputs=3
  Terminator{1..6} (6 alike) : Terminator
  vCf ph a  [V] : Outport
  iLf ph a [A] : Outport  Port=2
  iLoad pha [A] : Outport  Port=3
  "cos, sin" : Outport  Port=4
  wires:
  Demux1/3 -> Terminator4/1
  Demux/3 -> Terminator2/1
  Demux1/2 -> Terminator3/1
  Demux/2 -> Terminator1/1
  vCf [V]/1 -> Demux/1
  iLf [A]/1 -> Demux1/1
  Demux/1 -> vCf ph a  [V]/1
  Demux1/1 -> iLf ph a [A]/1
  Demux2/3 -> Terminator6/1
  Demux2/2 -> Terminator5/1
  iLoad [A]/1 -> Demux2/1
  Demux2/1 -> iLoad pha [A]/1
  cos sin/1 -> "cos, sin"/1

== system UPS_3level_Ttype_Inverter_simplified_ctrl/Output Inverter Control System SRF(dq0) - SPWM /SPWM (Treg)2/phase b signals ==
  vCf [V] : Inport
  iLf [A] : Inport  Port=2
  iLoad [A] : Inport  Port=3
  cos sin : Inport  Port=4
  Add : Sum
  Add1 : Sum
  Demux : Demux  Outputs=3
  Demux1 : Demux  Outputs=3
  Demux2 : Demux  Outputs=3
  Demux3 : Demux  Outputs=2
  Gain1 : Gain  Gain=cos(2*pi/3)
  Gain2 : Gain  Gain=sin(2*pi/3)
  Gain3 : Gain  Gain=cos(2*pi/3)
  Gain4 : Gain  Gain=-sin(2*pi/3)
  Mux2 : Mux  Inputs=2
  Terminator{1..6} (6 alike) : Terminator
  vCf ph b  [V] : Outport
  iLf ph b [A] : Outport  Port=2
  iLoad ph b [A] : Outport  Port=3
  cos sin rot -120 deg : Outport  Port=4
  wires:
  Demux1/2 -> iLf ph b [A]/1
  Demux/2 -> vCf ph b  [V]/1
  iLf [A]/1 -> Demux1/1
  vCf [V]/1 -> Demux/1
  Demux/1 -> Terminator1/1
  Demux1/1 -> Terminator3/1
  Demux/3 -> Terminator2/1
  Demux1/3 -> Terminator4/1
  Demux2/3 -> Terminator6/1
  Demux2/1 -> Terminator5/1
  cos sin/1 -> Demux3/1
  Demux3/1 -> Gain1/1, Gain4/1
  Demux3/2 -> Gain2/1, Gain3/1
  Gain1/1 -> Add/1
  Gain2/1 -> Add/2
  Add/1 -> Mux2/1
  Mux2/1 -> cos sin rot -120 deg/1
  Add1/1 -> Mux2/2
  Gain4/1 -> Add1/1
  Gain3/1 -> Add1/2
  iLoad [A]/1 -> Demux2/1
  Demux2/2 -> iLoad ph b [A]/1

== system UPS_3level_Ttype_Inverter_simplified_ctrl/Output Inverter Control System SRF(dq0) - SPWM /SPWM (Treg)2/phase c signals ==
  vCf [V] : Inport
  iLf [A] : Inport  Port=2
  iLoad [A] : Inport  Port=3
  cos sin : Inport  Port=4
  Add : Sum
  Add1 : Sum
  Demux : Demux  Outputs=3
  Demux1 : Demux  Outputs=3
  Demux2 : Demux  Outputs=3
  Demux3 : Demux  Outputs=2
  Gain1 : Gain  Gain=cos(2*pi/3)
  Gain2 : Gain  Gain=-sin(2*pi/3)
  Gain3 : Gain  Gain=cos(2*pi/3)
  Gain4 : Gain  Gain=sin(2*pi/3)
  Mux2 : Mux  Inputs=2
  Terminator{1..6} (6 alike) : Terminator
  vCf ph c  [V] : Outport
  iLf ph c [A] : Outport  Port=2
  iLoad ph c [A] : Outport  Port=3
  cos sin rot +120 deg : Outport  Port=4
  wires:
  Demux1/2 -> Terminator4/1
  Demux/2 -> Terminator2/1
  Demux1/1 -> Terminator3/1
  Demux/1 -> Terminator1/1
  vCf [V]/1 -> Demux/1
  iLf [A]/1 -> Demux1/1
  Demux/3 -> vCf ph c  [V]/1
  Demux1/3 -> iLf ph c [A]/1
  Demux2/1 -> Terminator6/1
  Demux2/2 -> Terminator5/1
  Gain3/1 -> Add1/2
  Gain4/1 -> Add1/1
  Add1/1 -> Mux2/2
  Mux2/1 -> cos sin rot +120 deg/1
  Add/1 -> Mux2/1
  Gain2/1 -> Add/2
  Gain1/1 -> Add/1
  Demux3/2 -> Gain3/1, Gain2/1
  Demux3/1 -> Gain4/1, Gain1/1
  cos sin/1 -> Demux3/1
  iLoad [A]/1 -> Demux2/1
  Demux2/3 -> iLoad ph c [A]/1

== system UPS_3level_Ttype_Inverter_simplified_ctrl/Output Inverter Control System SRF(dq0) - SPWM /SPWM (Treg)2/va, vb1 ==
  u [pu] : Inport
  Add : Sum  Inputs=+-
  Constant : Constant  Value=-1
  Constant1 : Constant
  Constant2 : Constant
  Data Type Conversion : DataTypeConversion  OutDataTypeStr=double
  Logical Operator : Logic  Operator=OR  AllPortsSameDT=off  OutDataTypeStr=boolean
  Relational Operator1 : RelationalOperator  Operator=<  OutDataTypeStr=boolean
  Relational Operator2 : RelationalOperator  Operator=>  OutDataTypeStr=boolean
  sat_comp : Outport
  wires:
  u [pu]/1 -> Relational Operator2/1, Relational Operator1/1
  Constant1/1 -> Relational Operator2/2
  Constant/1 -> Relational Operator1/2
  Relational Operator2/1 -> Logical Operator/1
  Relational Operator1/1 -> Logical Operator/2
  Logical Operator/1 -> Data Type Conversion/1
  Data Type Conversion/1 -> Add/2
  Add/1 -> sat_comp/1
  Constant2/1 -> Add/1

== system UPS_3level_Ttype_Inverter_simplified_ctrl/Output Inverter Control System SRF(dq0) - SPWM /SPWM (Treg)2/va, vb2 ==
  u [pu] : Inport
  Add : Sum  Inputs=+-
  Constant : Constant  Value=-1
  Constant1 : Constant
  Constant2 : Constant
  Data Type Conversion : DataTypeConversion  OutDataTypeStr=double
  Logical Operator : Logic  Operator=OR  AllPortsSameDT=off  OutDataTypeStr=boolean
  Relational Operator1 : RelationalOperator  Operator=<  OutDataTypeStr=boolean
  Relational Operator2 : RelationalOperator  Operator=>  OutDataTypeStr=boolean
  sat_comp : Outport
  wires:
  Constant2/1 -> Add/1
  Add/1 -> sat_comp/1
  Data Type Conversion/1 -> Add/2
  Logical Operator/1 -> Data Type Conversion/1
  Relational Operator1/1 -> Logical Operator/2
  Relational Operator2/1 -> Logical Operator/1
  Constant/1 -> Relational Operator1/2
  Constant1/1 -> Relational Operator2/2
  u [pu]/1 -> Relational Operator1/1, Relational Operator2/1

== system UPS_3level_Ttype_Inverter_simplified_ctrl/Output Inverter Control System SRF(dq0) - SPWM /SPWM (Treg)2/va, vb3 ==
  u [pu] : Inport
  Add : Sum  Inputs=+-
  Constant : Constant  Value=-1
  Constant1 : Constant
  Constant2 : Constant
  Data Type Conversion : DataTypeConversion  OutDataTypeStr=double
  Logical Operator : Logic  Operator=OR  AllPortsSameDT=off  OutDataTypeStr=boolean
  Relational Operator1 : RelationalOperator  Operator=<  OutDataTypeStr=boolean
  Relational Operator2 : RelationalOperator  Operator=>  OutDataTypeStr=boolean
  sat_comp : Outport
  wires:
  u [pu]/1 -> Relational Operator2/1, Relational Operator1/1
  Constant1/1 -> Relational Operator2/2
  Constant/1 -> Relational Operator1/2
  Relational Operator2/1 -> Logical Operator/1
  Relational Operator1/1 -> Logical Operator/2
  Logical Operator/1 -> Data Type Conversion/1
  Data Type Conversion/1 -> Add/2
  Add/1 -> sat_comp/1
  Constant2/1 -> Add/1

== system UPS_3level_Ttype_Inverter_simplified_ctrl/Output Inverter Control System SRF(dq0) - SPWM /SPWM (Treg)2/va, vb4 ==
  u [V] : Inport
  Vdcpn [V] : Inport  Port=2
  Demux : Demux  Outputs=2
  Divide1 : Product  Inputs=*/
  Gain : Gain  Gain=0.5
  Sum : Sum  Inputs=|++
  u [pu] : Outport
  wires:
  u [V]/1 -> Divide1/1
  Divide1/1 -> u [pu]/1
  Vdcpn [V]/1 -> Demux/1
  Demux/1 -> Sum/1
  Demux/2 -> Sum/2
  Sum/1 -> Gain/1
  Gain/1 -> Divide1/2

== system UPS_3level_Ttype_Inverter_simplified_ctrl/Output Inverter Control System SRF(dq0) - SPWM /SPWM (Treg)2/va, vb5 ==
  u [V] : Inport
  Vdcpn [V] : Inport  Port=2
  Demux : Demux  Outputs=2
  Divide1 : Product  Inputs=*/
  Gain : Gain  Gain=0.5
  Sum : Sum  Inputs=|++
  u [pu] : Outport
  wires:
  u [V]/1 -> Divide1/1
  Divide1/1 -> u [pu]/1
  Vdcpn [V]/1 -> Demux/1
  Demux/1 -> Sum/1
  Demux/2 -> Sum/2
  Sum/1 -> Gain/1
  Gain/1 -> Divide1/2

== system UPS_3level_Ttype_Inverter_simplified_ctrl/Output Inverter Control System SRF(dq0) - SPWM /SPWM (Treg)2/va, vb6 ==
  u [V] : Inport
  Vdcpn [V] : Inport  Port=2
  Demux : Demux  Outputs=2
  Divide1 : Product  Inputs=*/
  Gain : Gain  Gain=0.5
  Sum : Sum  Inputs=|++
  u [pu] : Outport
  wires:
  u [V]/1 -> Divide1/1
  Divide1/1 -> u [pu]/1
  Vdcpn [V]/1 -> Demux/1
  Demux/1 -> Sum/1
  Demux/2 -> Sum/2
  Sum/1 -> Gain/1
  Gain/1 -> Divide1/2

== system UPS_3level_Ttype_Inverter_simplified_ctrl/Output Inverter Control System SRF(dq0) - SPWM /3p PLL/va, vb/va* = Vm*cos(wrt)* ==
  Vm [pu] : Inport
  wrt [deg] : Inport  Port=2
  Fcn1 : Fcn  Expr=(cos(u(1)))
  Product : Product  SaturateOnIntegerOverflow=on  InputSameDT=on  OutDataTypeStr=Inherit: Same as first input
  d2r : Gain  Gain=pi/180  SaturateOnIntegerOverflow=on  OutDataTypeStr=Inherit: Same as input  ParamDataTypeStr=Inherit: Same as input
  va : Outport
  wires:
  d2r/1 -> Fcn1/1
  Fcn1/1 -> Product/1
  Vm [pu]/1 -> Product/2
  Product/1 -> va/1
  wrt [deg]/1 -> d2r/1

== system UPS_3level_Ttype_Inverter_simplified_ctrl/Output Inverter Control System SRF(dq0) - SPWM /3p PLL/va, vb/vb* = Vm*sin(wrt)* ==
  Vm [pu] : Inport
  wrt [deg] : Inport  Port=2
  Fcn1 : Fcn  Expr=(sin(u(1)))
  Product : Product  SaturateOnIntegerOverflow=on  InputSameDT=on  OutDataTypeStr=Inherit: Same as first input
  d2r : Gain  Gain=pi/180  SaturateOnIntegerOverflow=on  OutDataTypeStr=Inherit: Same as input  ParamDataTypeStr=Inherit: Same as input
  vb : Outport
  wires:
  d2r/1 -> Fcn1/1
  Fcn1/1 -> Product/1
  Vm [pu]/1 -> Product/2
  Product/1 -> vb/1
  wrt [deg]/1 -> d2r/1

== system UPS_3level_Ttype_Inverter_simplified_ctrl/Output Inverter Control System SRF(dq0) - SPWM /SPWM (Treg)2/ ADC System (Tinp//2)/ADC1 ==
  A : Inport
  Add1 : Sum  Inputs=+-
  Add2 : Sum
  Add3 : Sum
  Add7 : Sum
  Constant1 : Constant  Value=ADC.Voffset
  Constant2 : Constant  Value=(2^ADC.N)/2
  Data Type Conversion1 : DataTypeConversion  OutDataTypeStr=int16  SaturateOnIntegerOverflow=on  RndMeth=Zero
  Data Type Conversion2 : DataTypeConversion  OutDataTypeStr=double  SaturateOnIntegerOverflow=on  RndMeth=Zero
  Gain : Gain  Gain=ADC.k1vABC
  Gain1 : Gain  Gain=ADC.k2vABC
  Gain2 : Gain  Gain=ADC.Nonlin*((ADC.Vmax - ADC.Vmin)/2^ADC.N)
  Gain3 : Gain  Gain=ADC.Nnoise*((ADC.Vmax - ADC.Vmin)/2^ADC.N)
  Idealized ADC quantizer : simulink_extras/Additional Discrete/Idealized ADC quantizer  NumberOfConverterBits=ADC.N  Vmin=ADC.Vmin  Vmax=ADC.Vmax  OutputDataType=int16  OutputNegativeValues=off
  Uniform Random Number : UniformRandomNumber
  Uniform Random Number1 : UniformRandomNumber
  D : Outport
  wires:
  Gain/1 -> Add7/1
  Constant1/1 -> Add7/2
  Constant2/1 -> Data Type Conversion1/1
  Data Type Conversion1/1 -> Add1/2
  Idealized ADC quantizer/1 -> Add1/1
  A/1 -> Gain/1
  Gain1/1 -> D/1
  Add1/1 -> Data Type Conversion2/1
  Data Type Conversion2/1 -> Gain1/1
  Uniform Random Number/1 -> Gain2/1
  Gain2/1 -> Add2/2
  Uniform Random Number1/1 -> Gain3/1
  Gain3/1 -> Add3/2
  Add7/1 -> Add3/1
  Add3/1 -> Add2/1
  Add2/1 -> Idealized ADC quantizer/1

== system UPS_3level_Ttype_Inverter_simplified_ctrl/Output Inverter Control System SRF(dq0) - SPWM /SPWM (Treg)2/ ADC System (Tinp//2)/ADC10 ==
  A : Inport
  Add1 : Sum  Inputs=+-
  Add2 : Sum
  Add3 : Sum
  Add7 : Sum
  Constant1 : Constant  Value=ADC.Voffset
  Constant2 : Constant  Value=(2^ADC.N)/2
  Data Type Conversion1 : DataTypeConversion  OutDataTypeStr=int16  SaturateOnIntegerOverflow=on  RndMeth=Zero
  Data Type Conversion2 : DataTypeConversion  OutDataTypeStr=double  SaturateOnIntegerOverflow=on  RndMeth=Zero
  Gain : Gain  Gain=ADC.k1vDCpn
  Gain1 : Gain  Gain=ADC.k2vDCpn
  Gain2 : Gain  Gain=ADC.Nonlin*((ADC.Vmax - ADC.Vmin)/2^ADC.N)
  Gain3 : Gain  Gain=ADC.Nnoise*((ADC.Vmax - ADC.Vmin)/2^ADC.N)
  Idealized ADC quantizer : simulink_extras/Additional Discrete/Idealized ADC quantizer  NumberOfConverterBits=ADC.N  Vmin=ADC.Vmin  Vmax=ADC.Vmax  OutputDataType=int16  OutputNegativeValues=off
  Uniform Random Number : UniformRandomNumber
  Uniform Random Number1 : UniformRandomNumber
  D : Outport
  wires:
  Add3/1 -> Add2/1
  Add7/1 -> Add3/1
  Gain3/1 -> Add3/2
  Uniform Random Number1/1 -> Gain3/1
  Gain2/1 -> Add2/2
  Add2/1 -> Idealized ADC quantizer/1
  Uniform Random Number/1 -> Gain2/1
  Gain1/1 -> D/1
  Data Type Conversion2/1 -> Gain1/1
  Add1/1 -> Data Type Conversion2/1
  A/1 -> Gain/1
  Idealized ADC quantizer/1 -> Add1/1
  Data Type Conversion1/1 -> Add1/2
  Constant2/1 -> Data Type Conversion1/1
  Constant1/1 -> Add7/2
  Gain/1 -> Add7/1

== system UPS_3level_Ttype_Inverter_simplified_ctrl/Output Inverter Control System SRF(dq0) - SPWM /SPWM (Treg)2/ ADC System (Tinp//2)/ADC11 ==
  A : Inport
  Add1 : Sum  Inputs=+-
  Add2 : Sum
  Add3 : Sum
  Add7 : Sum
  Constant1 : Constant  Value=ADC.Voffset
  Constant2 : Constant  Value=(2^ADC.N)/2
  Data Type Conversion1 : DataTypeConversion  OutDataTypeStr=int16  SaturateOnIntegerOverflow=on  RndMeth=Zero
  Data Type Conversion2 : DataTypeConversion  OutDataTypeStr=double  SaturateOnIntegerOverflow=on  RndMeth=Zero
  Gain : Gain  Gain=ADC.k1vDCpn
  Gain1 : Gain  Gain=ADC.k2vDCpn
  Gain2 : Gain  Gain=ADC.Nonlin*((ADC.Vmax - ADC.Vmin)/2^ADC.N)
  Gain3 : Gain  Gain=ADC.Nnoise*((ADC.Vmax - ADC.Vmin)/2^ADC.N)
  Idealized ADC quantizer : simulink_extras/Additional Discrete/Idealized ADC quantizer  NumberOfConverterBits=ADC.N  Vmin=ADC.Vmin  Vmax=ADC.Vmax  OutputDataType=int16  OutputNegativeValues=off
  Uniform Random Number : UniformRandomNumber
  Uniform Random Number1 : UniformRandomNumber
  D : Outport
  wires:
  Gain/1 -> Add7/1
  Constant1/1 -> Add7/2
  Constant2/1 -> Data Type Conversion1/1
  Data Type Conversion1/1 -> Add1/2
  Idealized ADC quantizer/1 -> Add1/1
  A/1 -> Gain/1
  Add1/1 -> Data Type Conversion2/1
  Data Type Conversion2/1 -> Gain1/1
  Gain1/1 -> D/1
  Uniform Random Number/1 -> Gain2/1
  Add2/1 -> Idealized ADC quantizer/1
  Gain2/1 -> Add2/2
  Uniform Random Number1/1 -> Gain3/1
  Gain3/1 -> Add3/2
  Add7/1 -> Add3/1
  Add3/1 -> Add2/1

== system UPS_3level_Ttype_Inverter_simplified_ctrl/Output Inverter Control System SRF(dq0) - SPWM /SPWM (Treg)2/ ADC System (Tinp//2)/ADC2 ==
  A : Inport
  Add1 : Sum  Inputs=+-
  Add2 : Sum
  Add3 : Sum
  Add7 : Sum
  Constant1 : Constant  Value=ADC.Voffset
  Constant2 : Constant  Value=(2^ADC.N)/2
  Data Type Conversion1 : DataTypeConversion  OutDataTypeStr=int16  SaturateOnIntegerOverflow=on  RndMeth=Zero
  Data Type Conversion2 : DataTypeConversion  OutDataTypeStr=double  SaturateOnIntegerOverflow=on  RndMeth=Zero
  Gain : Gain  Gain=ADC.k1vABC
  Gain1 : Gain  Gain=ADC.k2vABC
  Gain2 : Gain  Gain=ADC.Nonlin*((ADC.Vmax - ADC.Vmin)/2^ADC.N)
  Gain3 : Gain  Gain=ADC.Nnoise*((ADC.Vmax - ADC.Vmin)/2^ADC.N)
  Idealized ADC quantizer : simulink_extras/Additional Discrete/Idealized ADC quantizer  NumberOfConverterBits=ADC.N  Vmin=ADC.Vmin  Vmax=ADC.Vmax  OutputDataType=int16  OutputNegativeValues=off
  Uniform Random Number : UniformRandomNumber
  Uniform Random Number1 : UniformRandomNumber
  D : Outport
  wires:
  Gain/1 -> Add7/1
  Constant1/1 -> Add7/2
  Constant2/1 -> Data Type Conversion1/1
  Data Type Conversion1/1 -> Add1/2
  Idealized ADC quantizer/1 -> Add1/1
  A/1 -> Gain/1
  Gain1/1 -> D/1
  Add1/1 -> Data Type Conversion2/1
  Data Type Conversion2/1 -> Gain1/1
  Add2/1 -> Idealized ADC quantizer/1
  Uniform Random Number/1 -> Gain2/1
  Gain2/1 -> Add2/2
  Uniform Random Number1/1 -> Gain3/1
  Gain3/1 -> Add3/2
  Add7/1 -> Add3/1
  Add3/1 -> Add2/1

== system UPS_3level_Ttype_Inverter_simplified_ctrl/Output Inverter Control System SRF(dq0) - SPWM /SPWM (Treg)2/ ADC System (Tinp//2)/ADC3 ==
  A : Inport
  Add1 : Sum  Inputs=+-
  Add2 : Sum
  Add3 : Sum
  Add7 : Sum
  Constant1 : Constant  Value=ADC.Voffset
  Constant2 : Constant  Value=(2^ADC.N)/2
  Data Type Conversion1 : DataTypeConversion  OutDataTypeStr=int16  SaturateOnIntegerOverflow=on  RndMeth=Zero
  Data Type Conversion2 : DataTypeConversion  OutDataTypeStr=double  SaturateOnIntegerOverflow=on  RndMeth=Zero
  Gain : Gain  Gain=ADC.k1vABC
  Gain1 : Gain  Gain=ADC.k2vABC
  Gain2 : Gain  Gain=ADC.Nonlin*((ADC.Vmax - ADC.Vmin)/2^ADC.N)
  Gain3 : Gain  Gain=ADC.Nnoise*((ADC.Vmax - ADC.Vmin)/2^ADC.N)
  Idealized ADC quantizer : simulink_extras/Additional Discrete/Idealized ADC quantizer  NumberOfConverterBits=ADC.N  Vmin=ADC.Vmin  Vmax=ADC.Vmax  OutputDataType=int16  OutputNegativeValues=off
  Uniform Random Number : UniformRandomNumber
  Uniform Random Number1 : UniformRandomNumber
  D : Outport
  wires:
  Gain/1 -> Add7/1
  Constant1/1 -> Add7/2
  Constant2/1 -> Data Type Conversion1/1
  Data Type Conversion1/1 -> Add1/2
  Idealized ADC quantizer/1 -> Add1/1
  A/1 -> Gain/1
  Gain1/1 -> D/1
  Add1/1 -> Data Type Conversion2/1
  Data Type Conversion2/1 -> Gain1/1
  Uniform Random Number/1 -> Gain2/1
  Gain2/1 -> Add2/2
  Uniform Random Number1/1 -> Gain3/1
  Gain3/1 -> Add3/2
  Add7/1 -> Add3/1
  Add3/1 -> Add2/1
  Add2/1 -> Idealized ADC quantizer/1

== system UPS_3level_Ttype_Inverter_simplified_ctrl/Output Inverter Control System SRF(dq0) - SPWM /SPWM (Treg)2/ ADC System (Tinp//2)/ADC4 ==
  A : Inport
  Add1 : Sum  Inputs=+-
  Add2 : Sum
  Add3 : Sum
  Add7 : Sum
  Constant1 : Constant  Value=ADC.Voffset
  Constant2 : Constant  Value=(2^ADC.N)/2
  Data Type Conversion1 : DataTypeConversion  OutDataTypeStr=int16  SaturateOnIntegerOverflow=on  RndMeth=Zero
  Data Type Conversion2 : DataTypeConversion  OutDataTypeStr=double  SaturateOnIntegerOverflow=on  RndMeth=Zero
  Gain : Gain  Gain=ADC.k1iABC
  Gain1 : Gain  Gain=ADC.k2iABC
  Gain2 : Gain  Gain=ADC.Nonlin*((ADC.Vmax - ADC.Vmin)/2^ADC.N)
  Gain3 : Gain  Gain=ADC.Nnoise*((ADC.Vmax - ADC.Vmin)/2^ADC.N)
  Idealized ADC quantizer : simulink_extras/Additional Discrete/Idealized ADC quantizer  NumberOfConverterBits=ADC.N  Vmin=ADC.Vmin  Vmax=ADC.Vmax  OutputDataType=int16  OutputNegativeValues=off
  Uniform Random Number : UniformRandomNumber
  Uniform Random Number1 : UniformRandomNumber
  D : Outport
  wires:
  Gain/1 -> Add7/1
  Constant1/1 -> Add7/2
  Constant2/1 -> Data Type Conversion1/1
  Data Type Conversion1/1 -> Add1/2
  Idealized ADC quantizer/1 -> Add1/1
  A/1 -> Gain/1
  Gain1/1 -> D/1
  Add1/1 -> Data Type Conversion2/1
  Data Type Conversion2/1 -> Gain1/1
  Add2/1 -> Idealized ADC quantizer/1
  Uniform Random Number/1 -> Gain2/1
  Gain2/1 -> Add2/2
  Uniform Random Number1/1 -> Gain3/1
  Gain3/1 -> Add3/2
  Add7/1 -> Add3/1
  Add3/1 -> Add2/1

== system UPS_3level_Ttype_Inverter_simplified_ctrl/Output Inverter Control System SRF(dq0) - SPWM /SPWM (Treg)2/ ADC System (Tinp//2)/ADC5 ==
  A : Inport
  Add1 : Sum  Inputs=+-
  Add2 : Sum
  Add3 : Sum
  Add7 : Sum
  Constant1 : Constant  Value=ADC.Voffset
  Constant2 : Constant  Value=(2^ADC.N)/2
  Data Type Conversion1 : DataTypeConversion  OutDataTypeStr=int16  SaturateOnIntegerOverflow=on  RndMeth=Zero
  Data Type Conversion2 : DataTypeConversion  OutDataTypeStr=double  SaturateOnIntegerOverflow=on  RndMeth=Zero
  Gain : Gain  Gain=ADC.k1iABC
  Gain1 : Gain  Gain=ADC.k2iABC
  Gain2 : Gain  Gain=ADC.Nonlin*((ADC.Vmax - ADC.Vmin)/2^ADC.N)
  Gain3 : Gain  Gain=ADC.Nnoise*((ADC.Vmax - ADC.Vmin)/2^ADC.N)
  Idealized ADC quantizer : simulink_extras/Additional Discrete/Idealized ADC quantizer  NumberOfConverterBits=ADC.N  Vmin=ADC.Vmin  Vmax=ADC.Vmax  OutputDataType=int16  OutputNegativeValues=off
  Uniform Random Number : UniformRandomNumber
  Uniform Random Number1 : UniformRandomNumber
  D : Outport
  wires:
  Gain/1 -> Add7/1
  Constant1/1 -> Add7/2
  Constant2/1 -> Data Type Conversion1/1
  Data Type Conversion1/1 -> Add1/2
  Idealized ADC quantizer/1 -> Add1/1
  A/1 -> Gain/1
  Gain1/1 -> D/1
  Add1/1 -> Data Type Conversion2/1
  Data Type Conversion2/1 -> Gain1/1
  Add2/1 -> Idealized ADC quantizer/1
  Uniform Random Number/1 -> Gain2/1
  Gain2/1 -> Add2/2
  Uniform Random Number1/1 -> Gain3/1
  Gain3/1 -> Add3/2
  Add7/1 -> Add3/1
  Add3/1 -> Add2/1

== system UPS_3level_Ttype_Inverter_simplified_ctrl/Output Inverter Control System SRF(dq0) - SPWM /SPWM (Treg)2/ ADC System (Tinp//2)/ADC6 ==
  A : Inport
  Add1 : Sum  Inputs=+-
  Add2 : Sum
  Add3 : Sum
  Add7 : Sum
  Constant1 : Constant  Value=ADC.Voffset
  Constant2 : Constant  Value=(2^ADC.N)/2
  Data Type Conversion1 : DataTypeConversion  OutDataTypeStr=int16  SaturateOnIntegerOverflow=on  RndMeth=Zero
  Data Type Conversion2 : DataTypeConversion  OutDataTypeStr=double  SaturateOnIntegerOverflow=on  RndMeth=Zero
  Gain : Gain  Gain=ADC.k1iABC
  Gain1 : Gain  Gain=ADC.k2iABC
  Gain2 : Gain  Gain=ADC.Nonlin*((ADC.Vmax - ADC.Vmin)/2^ADC.N)
  Gain3 : Gain  Gain=ADC.Nnoise*((ADC.Vmax - ADC.Vmin)/2^ADC.N)
  Idealized ADC quantizer : simulink_extras/Additional Discrete/Idealized ADC quantizer  NumberOfConverterBits=ADC.N  Vmin=ADC.Vmin  Vmax=ADC.Vmax  OutputDataType=int16  OutputNegativeValues=off
  Uniform Random Number : UniformRandomNumber
  Uniform Random Number1 : UniformRandomNumber
  D : Outport
  wires:
  Gain/1 -> Add7/1
  Constant1/1 -> Add7/2
  Constant2/1 -> Data Type Conversion1/1
  Data Type Conversion1/1 -> Add1/2
  Idealized ADC quantizer/1 -> Add1/1
  A/1 -> Gain/1
  Gain1/1 -> D/1
  Add1/1 -> Data Type Conversion2/1
  Data Type Conversion2/1 -> Gain1/1
  Add2/1 -> Idealized ADC quantizer/1
  Uniform Random Number/1 -> Gain2/1
  Gain2/1 -> Add2/2
  Uniform Random Number1/1 -> Gain3/1
  Gain3/1 -> Add3/2
  Add7/1 -> Add3/1
  Add3/1 -> Add2/1

== system UPS_3level_Ttype_Inverter_simplified_ctrl/Output Inverter Control System SRF(dq0) - SPWM /SPWM (Treg)2/ ADC System (Tinp//2)/ADC7 ==
  A : Inport
  Add1 : Sum  Inputs=+-
  Add2 : Sum
  Add3 : Sum
  Add7 : Sum
  Constant1 : Constant  Value=ADC.Voffset
  Constant2 : Constant  Value=(2^ADC.N)/2
  Data Type Conversion1 : DataTypeConversion  OutDataTypeStr=int16  SaturateOnIntegerOverflow=on  RndMeth=Zero
  Data Type Conversion2 : DataTypeConversion  OutDataTypeStr=double  SaturateOnIntegerOverflow=on  RndMeth=Zero
  Gain : Gain  Gain=ADC.k1iABC
  Gain1 : Gain  Gain=ADC.k2iABC
  Gain2 : Gain  Gain=ADC.Nonlin*((ADC.Vmax - ADC.Vmin)/2^ADC.N)
  Gain3 : Gain  Gain=ADC.Nnoise*((ADC.Vmax - ADC.Vmin)/2^ADC.N)
  Idealized ADC quantizer : simulink_extras/Additional Discrete/Idealized ADC quantizer  NumberOfConverterBits=ADC.N  Vmin=ADC.Vmin  Vmax=ADC.Vmax  OutputDataType=int16  OutputNegativeValues=off
  Uniform Random Number : UniformRandomNumber
  Uniform Random Number1 : UniformRandomNumber
  D : Outport
  wires:
  Gain/1 -> Add7/1
  Constant1/1 -> Add7/2
  Constant2/1 -> Data Type Conversion1/1
  Data Type Conversion1/1 -> Add1/2
  Idealized ADC quantizer/1 -> Add1/1
  A/1 -> Gain/1
  Gain1/1 -> D/1
  Add1/1 -> Data Type Conversion2/1
  Data Type Conversion2/1 -> Gain1/1
  Add2/1 -> Idealized ADC quantizer/1
  Uniform Random Number/1 -> Gain2/1
  Gain2/1 -> Add2/2
  Uniform Random Number1/1 -> Gain3/1
  Gain3/1 -> Add3/2
  Add7/1 -> Add3/1
  Add3/1 -> Add2/1

== system UPS_3level_Ttype_Inverter_simplified_ctrl/Output Inverter Control System SRF(dq0) - SPWM /SPWM (Treg)2/ ADC System (Tinp//2)/ADC8 ==
  A : Inport
  Add1 : Sum  Inputs=+-
  Add2 : Sum
  Add3 : Sum
  Add7 : Sum
  Constant1 : Constant  Value=ADC.Voffset
  Constant2 : Constant  Value=(2^ADC.N)/2
  Data Type Conversion1 : DataTypeConversion  OutDataTypeStr=int16  SaturateOnIntegerOverflow=on  RndMeth=Zero
  Data Type Conversion2 : DataTypeConversion  OutDataTypeStr=double  SaturateOnIntegerOverflow=on  RndMeth=Zero
  Gain : Gain  Gain=ADC.k1iABC
  Gain1 : Gain  Gain=ADC.k2iABC
  Gain2 : Gain  Gain=ADC.Nonlin*((ADC.Vmax - ADC.Vmin)/2^ADC.N)
  Gain3 : Gain  Gain=ADC.Nnoise*((ADC.Vmax - ADC.Vmin)/2^ADC.N)
  Idealized ADC quantizer : simulink_extras/Additional Discrete/Idealized ADC quantizer  NumberOfConverterBits=ADC.N  Vmin=ADC.Vmin  Vmax=ADC.Vmax  OutputDataType=int16  OutputNegativeValues=off
  Uniform Random Number : UniformRandomNumber
  Uniform Random Number1 : UniformRandomNumber
  D : Outport
  wires:
  Gain/1 -> Add7/1
  Constant1/1 -> Add7/2
  Constant2/1 -> Data Type Conversion1/1
  Data Type Conversion1/1 -> Add1/2
  Idealized ADC quantizer/1 -> Add1/1
  A/1 -> Gain/1
  Gain1/1 -> D/1
  Add1/1 -> Data Type Conversion2/1
  Data Type Conversion2/1 -> Gain1/1
  Add2/1 -> Idealized ADC quantizer/1
  Uniform Random Number/1 -> Gain2/1
  Gain2/1 -> Add2/2
  Uniform Random Number1/1 -> Gain3/1
  Gain3/1 -> Add3/2
  Add7/1 -> Add3/1
  Add3/1 -> Add2/1

== system UPS_3level_Ttype_Inverter_simplified_ctrl/Output Inverter Control System SRF(dq0) - SPWM /SPWM (Treg)2/ ADC System (Tinp//2)/ADC9 ==
  A : Inport
  Add1 : Sum  Inputs=+-
  Add2 : Sum
  Add3 : Sum
  Add7 : Sum
  Constant1 : Constant  Value=ADC.Voffset
  Constant2 : Constant  Value=(2^ADC.N)/2
  Data Type Conversion1 : DataTypeConversion  OutDataTypeStr=int16  SaturateOnIntegerOverflow=on  RndMeth=Zero
  Data Type Conversion2 : DataTypeConversion  OutDataTypeStr=double  SaturateOnIntegerOverflow=on  RndMeth=Zero
  Gain : Gain  Gain=ADC.k1iABC
  Gain1 : Gain  Gain=ADC.k2iABC
  Gain2 : Gain  Gain=ADC.Nonlin*((ADC.Vmax - ADC.Vmin)/2^ADC.N)
  Gain3 : Gain  Gain=ADC.Nnoise*((ADC.Vmax - ADC.Vmin)/2^ADC.N)
  Idealized ADC quantizer : simulink_extras/Additional Discrete/Idealized ADC quantizer  NumberOfConverterBits=ADC.N  Vmin=ADC.Vmin  Vmax=ADC.Vmax  OutputDataType=int16  OutputNegativeValues=off
  Uniform Random Number : UniformRandomNumber
  Uniform Random Number1 : UniformRandomNumber
  D : Outport
  wires:
  Gain/1 -> Add7/1
  Constant1/1 -> Add7/2
  Constant2/1 -> Data Type Conversion1/1
  Data Type Conversion1/1 -> Add1/2
  Idealized ADC quantizer/1 -> Add1/1
  A/1 -> Gain/1
  Gain1/1 -> D/1
  Add1/1 -> Data Type Conversion2/1
  Data Type Conversion2/1 -> Gain1/1
  Uniform Random Number/1 -> Gain2/1
  Gain2/1 -> Add2/2
  Uniform Random Number1/1 -> Gain3/1
  Gain3/1 -> Add3/2
  Add7/1 -> Add3/1
  Add3/1 -> Add2/1
  Add2/1 -> Idealized ADC quantizer/1

== system UPS_3level_Ttype_Inverter_simplified_ctrl/Output Inverter Control System SRF(dq0) - SPWM /SPWM (Treg)2/controller ph a1/Kalman Estimation fundamental ==
  iLoad [A] : Inport
  Demux2 : Demux  Outputs=2
  Discrete State-Space4 : DiscreteStateSpace  A=CTRL.AKd2  B=CTRL.BKd2  C=CTRL.CKd2  D=CTRL.DKd2  X0=[0;0]  SampleTime=-1
  iLoad_est cos [A] : Outport
  iLoad_est sin [A] : Outport  Port=2
  wires:
  iLoad [A]/1 -> Discrete State-Space4/1
  Discrete State-Space4/1 -> Demux2/1
  Demux2/1 -> iLoad_est cos [A]/1
  Demux2/2 -> iLoad_est sin [A]/1

== system UPS_3level_Ttype_Inverter_simplified_ctrl/Output Inverter Control System SRF(dq0) - SPWM /SPWM (Treg)2/controller ph a1/LQR gain ==
  iLf error [A] : Inport
  vCf error [V] : Inport  Port=2
  Add3 : Sum
  Gain : Gain  Gain=CTRL.Klq(1)
  Gain3 : Gain  Gain=CTRL.Klq(2)
  delta u [V] : Outport
  wires:
  Gain3/1 -> Add3/2
  Gain/1 -> Add3/1
  vCf error [V]/1 -> Gain3/1
  iLf error [A]/1 -> Gain/1
  Add3/1 -> delta u [V]/1
